simulink model "DSRCDOB"  (R2021a)
settings: Solver=VariableStepAuto  StartTime=0.0  StopTime=15.0  RelTol=1e-3
undefined symbols (not defined in the file): a, alpha, betac, delay, delay_a, gnet, omega
libraries: simulink x1
settings Model: Creator=shiva  LastModifiedBy=shiva

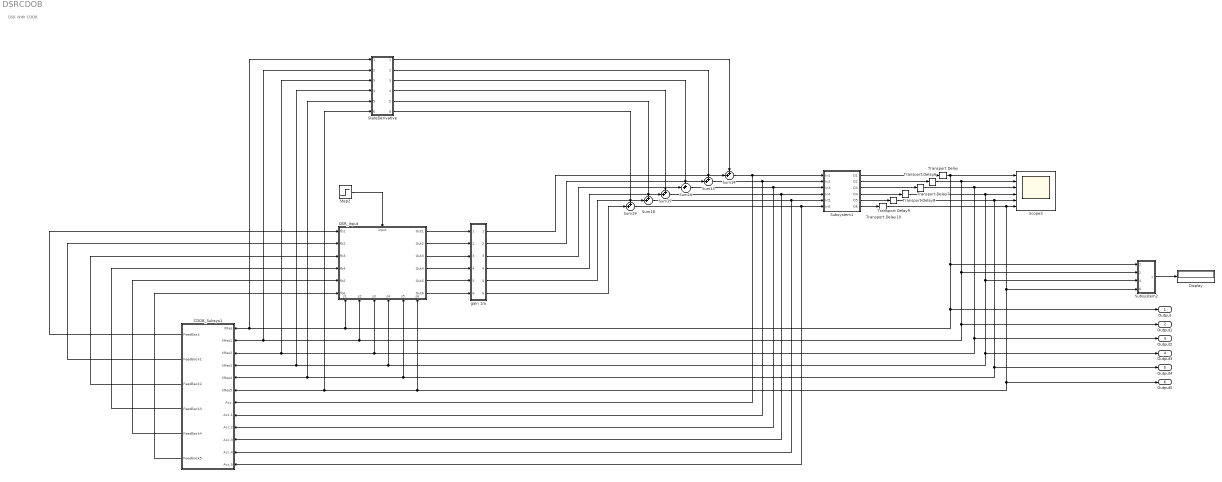
== system DSRCDOB ==
  note: DSR With CDOB
  CDOB_Subsys1 : Subsystem
  DSR_Input : Subsystem
      settings: PortSchema="{\"entries\":[{\"content\":{\"sides\":[{\"content\":{\"connectorIds\":[\"In1\",\"In2\",\"In3\",\"In4\",\"In5\",\"In6\"]},\"type\":\"ConnectorPlacement.EquallySpacedRectSide\",\"uuid\":\"7b8a38d4-2828-429e-a347-8750a0874c90\"},{\"content\":{\"connectorIds\":[\"Out1\",\"Out2\",\"Out3\",\"Out4\",\"Out5\",\"Out6\"],\"side\":\"RIGHT\"},\"type\":\"ConnectorPlacement.EquallySpacedRectSide\",\"uuid\":\"f1dcdaa7-0a93-43e2-be3b-ce942cee3b23\"},{\"content\":{\"connectorIds\":[\"In7\"],\"side\":\"TOP\"},\"type\":\"ConnectorPlacement.EquallySpacedRectSide\",\"uuid\":\"691a82b2-07cc-468b-b9a0-c0927a09fa47\"},{\"content\":{\"connectorIds\":[\"In8\",\"In9\",\"In10\",\"In11\",\"In12\",\"In13\"],\"side\":\"BOTTOM\"},\"type\":\"ConnectorPlacement.EquallySpacedRectSide\",\"uuid\":\"87ba8582-7e13-41cf-953e-972bab5f6463\"}]},\"type\":\"ConnectorPlacement.EquallySpacedConnector\",\"uuid\":\"6089c568-97aa-4e95-8448-5d1116d5973e\"}],\"packageUris\":[\"http://schema.mathworks.com/mf0/Connector/R2020b\"],\"version\":\"1.0\"}"
  Display : Display
  Scope3 : Scope  NumInputPorts=6
  StateDerivative : Subsystem
  Step2 : Step  Time=0  SampleTime=0
  Subsystem1 : Subsystem
  Subsystem2 : Subsystem
  Sum{14..19} (6 alike) : Sum  Inputs=++|
  Transport Delay{,6..10} (6 alike) : TransportDelay  DelayTime=delay_a
  gain 1/a : Subsystem
  Output : Outport
  Output1 : Outport  Port=2
  Output2 : Outport  Port=3
  Output3 : Outport  Port=4
  Output4 : Outport  Port=5
  Output5 : Outport  Port=6
  wires:
  Sum17/1 -> CDOB_Subsys1/10(Acc.3), Subsystem1/4(In4)
  Subsystem1/3(O3) -> Transport Delay7/1
  Step2/1 -> DSR_Input/7(input)
  Subsystem1/2(O2) -> Transport Delay6/1
  StateDerivative/5(Out5) -> Sum18/1
  StateDerivative/6(Out6) -> Sum19/1
  StateDerivative/1(Out1) -> Sum14/1
  StateDerivative/3(Out3) -> Sum16/1
  gain 1/a/1(Out1) -> Sum14/2
  Transport Delay6/1 -> Subsystem2/2(Input1), Output1/1, DSR_Input/9(s2), StateDerivative/2(Input1), CDOB_Subsys1/2(XRes1), Scope3/2
  DSR_Input/3(Out3) -> gain 1/a/3(In3)
  Transport Delay7/1 -> Output2/1, DSR_Input/10(s3), StateDerivative/3(Input2), CDOB_Subsys1/3(XRes2), Scope3/3
  CDOB_Subsys1/1(FeedBack) -> DSR_Input/1(fb1)
  Subsystem1/1(O1) -> Transport Delay/1
  Sum18/1 -> CDOB_Subsys1/11(Acc.4), Subsystem1/5(In5)
  DSR_Input/5(Out5) -> gain 1/a/5(In5)
  gain 1/a/4(Out4) -> Sum17/2
  CDOB_Subsys1/4(FeedBack3) -> DSR_Input/4(fb4)
  Transport Delay9/1 -> Output4/1, DSR_Input/12(s5), StateDerivative/5(Input4), CDOB_Subsys1/5(XRes4), Scope3/5
  Subsystem1/6(O6) -> Transport Delay10/1
  CDOB_Subsys1/2(FeedBack1) -> DSR_Input/2(fb2)
  DSR_Input/2(Out2) -> gain 1/a/2(In2)
  gain 1/a/2(Out2) -> Sum15/2
  CDOB_Subsys1/5(FeedBack4) -> DSR_Input/5(fb5)
  CDOB_Subsys1/3(FeedBack2) -> DSR_Input/3(fb3)
  Transport Delay10/1 -> Subsystem2/4(6), Output5/1, DSR_Input/13(s6), StateDerivative/6(Input5), CDOB_Subsys1/6(XRes5), Scope3/6
  StateDerivative/2(Out2) -> Sum15/1
  DSR_Input/4(Out4) -> gain 1/a/4(In4)
  DSR_Input/1(Out1) -> gain 1/a/1(In1)
  gain 1/a/3(Out3) -> Sum16/2
  Sum15/1 -> CDOB_Subsys1/8(Acc.1), Subsystem1/2(In2)
  DSR_Input/6(Out6) -> gain 1/a/6(In6)
  Subsystem1/5(O5) -> Transport Delay9/1
  gain 1/a/5(Out5) -> Sum18/2
  gain 1/a/6(Out6) -> Sum19/2
  StateDerivative/4(Out4) -> Sum17/1
  Transport Delay8/1 -> Subsystem2/3(4), Output3/1, DSR_Input/11(s4), StateDerivative/4(Input3), CDOB_Subsys1/4(XRes3), Scope3/4
  Subsystem1/4(O4) -> Transport Delay8/1
  Sum19/1 -> CDOB_Subsys1/12(Acc.5), Subsystem1/6(In6)
  Sum16/1 -> CDOB_Subsys1/9(Acc.2), Subsystem1/3(In3)
  Subsystem2/1(y) -> Display/1
  Sum14/1 -> CDOB_Subsys1/7(Acc.), Subsystem1/1(In1)
  CDOB_Subsys1/6(FeedBack5) -> DSR_Input/6(fb6)
  Transport Delay/1 -> Scope3/1, Subsystem2/1(Input), Output/1, DSR_Input/8(s1), StateDerivative/1(Input), CDOB_Subsys1/1(XRes)

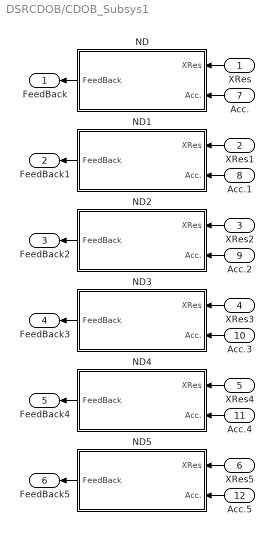
== system DSRCDOB/CDOB_Subsys1 ==
  XRes : Inport
  XRes1 : Inport  Port=2
  XRes2 : Inport  Port=3
  XRes3 : Inport  Port=4
  XRes4 : Inport  Port=5
  XRes5 : Inport  Port=6
  Acc. : Inport  Port=7
  Acc.1 : Inport  Port=8
  Acc.2 : Inport  Port=9
  Acc.3 : Inport  Port=10
  Acc.4 : Inport  Port=11
  Acc.5 : Inport  Port=12
  ND : Subsystem
  ND1 : Subsystem
  ND2 : Subsystem
  ND3 : Subsystem
  ND4 : Subsystem
  ND5 : Subsystem
  FeedBack : Outport
  FeedBack1 : Outport  Port=2
  FeedBack2 : Outport  Port=3
  FeedBack3 : Outport  Port=4
  FeedBack4 : Outport  Port=5
  FeedBack5 : Outport  Port=6
  wires:
  Acc./1 -> ND/2(Acc.)
  XRes/1 -> ND/1(XRes)
  Acc.4/1 -> ND4/2(Acc.)
  Acc.3/1 -> ND3/2(Acc.)
  XRes1/1 -> ND1/1(XRes)
  XRes2/1 -> ND2/1(XRes)
  XRes4/1 -> ND4/1(XRes)
  XRes5/1 -> ND5/1(XRes)
  Acc.2/1 -> ND2/2(Acc.)
  ND5/1(FeedBack) -> FeedBack5/1
  ND1/1(FeedBack) -> FeedBack1/1
  ND2/1(FeedBack) -> FeedBack2/1
  Acc.5/1 -> ND5/2(Acc.)
  ND4/1(FeedBack) -> FeedBack4/1
  ND/1(FeedBack) -> FeedBack/1
  ND3/1(FeedBack) -> FeedBack3/1
  XRes3/1 -> ND3/1(XRes)
  Acc.1/1 -> ND1/2(Acc.)

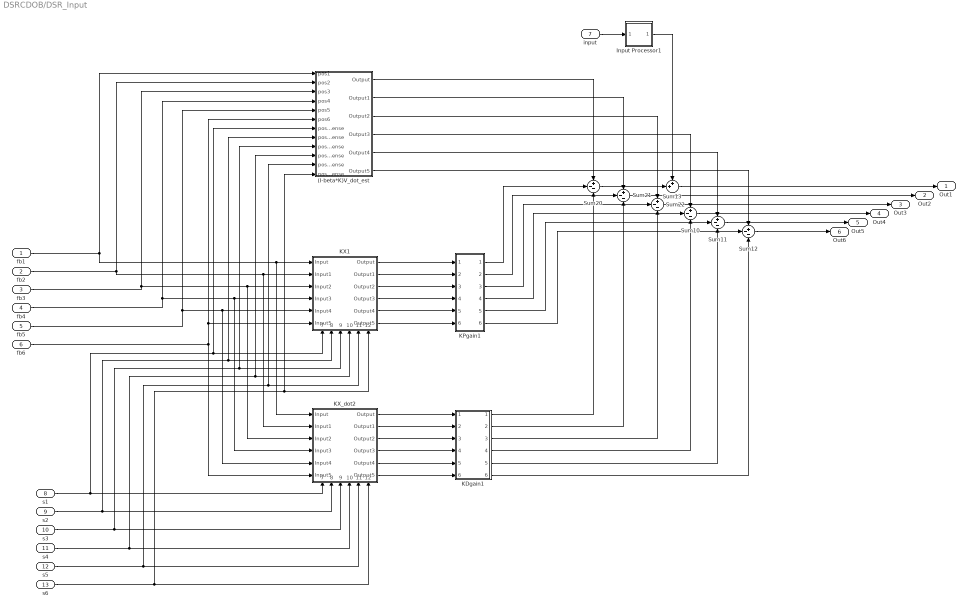
== system DSRCDOB/DSR_Input ==
  fb1 : Inport
  fb2 : Inport  Port=2
  fb3 : Inport  Port=3
  fb4 : Inport  Port=4
  fb5 : Inport  Port=5
  fb6 : Inport  Port=6
  input : Inport  Port=7
  s1 : Inport  Port=8
  s2 : Inport  Port=9
  s3 : Inport  Port=10
  s4 : Inport  Port=11
  s5 : Inport  Port=12
  s6 : Inport  Port=13
  (I-beta*K)V_dot_est : Subsystem
  Input Processor1 : Subsystem
  KDgain1 : Subsystem
  KPgain1 : Subsystem
  KX1 : Subsystem
      settings: PortSchema="{\"entries\":[{\"content\":{\"sides\":[{\"content\":{\"connectorIds\":[\"In1\",\"In2\",\"In3\",\"In4\",\"In5\",\"In6\"]},\"type\":\"ConnectorPlacement.EquallySpacedRectSide\",\"uuid\":\"24ff0189-2e26-4de2-9c90-2043606e3d63\"},{\"content\":{\"connectorIds\":[\"Out1\",\"Out2\",\"Out3\",\"Out4\",\"Out5\",\"Out6\"],\"side\":\"RIGHT\"},\"type\":\"ConnectorPlacement.EquallySpacedRectSide\",\"uuid\":\"7efe01dd-8101-429e-adc6-a10b45356e48\"},{\"content\":{\"connectorIds\":[],\"side\":\"TOP\"},\"type\":\"ConnectorPlacement.EquallySpacedRectSide\",\"uuid\":\"5c1fc1f4-b8b0-4afd-80fe-11f4d157d0fc\"},{\"content\":{\"connectorIds\":[\"In7\",\"In8\",\"In9\",\"In10\",\"In11\",\"In12\"],\"side\":\"BOTTOM\"},\"type\":\"ConnectorPlacement.EquallySpacedRectSide\",\"uuid\":\"e52c51d8-b236-4cc8-9958-a8d91e3741c4\"}]},\"type\":\"ConnectorPlacement.EquallySpacedConnector\",\"uuid\":\"3e3502e3-b8a3-4e9d-9b78-ab08dd870d4b\"}],\"packageUris\":[\"http://schema.mathworks.com/mf0/Connector/R2020b\"],\"version\":\"1.0\"}"
  KX_dot2 : Subsystem
      settings: PortSchema="{\"entries\":[{\"content\":{\"sides\":[{\"content\":{\"connectorIds\":[\"In1\",\"In2\",\"In3\",\"In4\",\"In5\",\"In6\"]},\"type\":\"ConnectorPlacement.EquallySpacedRectSide\",\"uuid\":\"24ff0189-2e26-4de2-9c90-2043606e3d63\"},{\"content\":{\"connectorIds\":[\"Out1\",\"Out2\",\"Out3\",\"Out4\",\"Out5\",\"Out6\"],\"side\":\"RIGHT\"},\"type\":\"ConnectorPlacement.EquallySpacedRectSide\",\"uuid\":\"7efe01dd-8101-429e-adc6-a10b45356e48\"},{\"content\":{\"connectorIds\":[],\"side\":\"TOP\"},\"type\":\"ConnectorPlacement.EquallySpacedRectSide\",\"uuid\":\"5c1fc1f4-b8b0-4afd-80fe-11f4d157d0fc\"},{\"content\":{\"connectorIds\":[\"In7\",\"In8\",\"In9\",\"In10\",\"In11\",\"In12\"],\"side\":\"BOTTOM\"},\"type\":\"ConnectorPlacement.EquallySpacedRectSide\",\"uuid\":\"bae418dc-ca78-4370-85bb-31cb43009c14\"}]},\"type\":\"ConnectorPlacement.EquallySpacedConnector\",\"uuid\":\"3e3502e3-b8a3-4e9d-9b78-ab08dd870d4b\"}],\"packageUris\":[\"http://schema.mathworks.com/mf0/Connector/R2020b\"],\"version\":\"1.0\"}"
  Sum{10..12,20..22} (6 alike) : Sum  Inputs=+--
  Sum13 : Sum  Inputs=++|
  Out1 : Outport
  Out2 : Outport  Port=2
  Out3 : Outport  Port=3
  Out4 : Outport  Port=4
  Out5 : Outport  Port=5
  Out6 : Outport  Port=6
  wires:
  KX_dot2/5(Output4) -> KDgain1/5(Output4)
  fb4/1 -> KX1/4(Input3), KX_dot2/4(Input3), (I-beta*K)V_dot_est/4(pos4)
  fb2/1 -> KX1/2(Input1), KX_dot2/2(Input1), (I-beta*K)V_dot_est/2(pos2)
  KDgain1/6(Out6) -> Sum12/3
  fb3/1 -> KX1/3(Input2), KX_dot2/3(Input2), (I-beta*K)V_dot_est/3(pos3)
  KPgain1/4(Out4) -> Sum10/2
  Sum10/1 -> Out4/1
  KPgain1/2(Out2) -> Sum21/2
  KX1/6(Output5) -> KPgain1/6(Output5)
  KX1/2(Output1) -> KPgain1/2(Output1)
  KPgain1/6(Out6) -> Sum12/2
  KX1/4(Output3) -> KPgain1/4(Output3)
  KX1/3(Output2) -> KPgain1/3(Output2)
  s6/1 -> KX_dot2/12(sense6), (I-beta*K)V_dot_est/12(pos6sense), KX1/12(sense6)
  KDgain1/4(Out4) -> Sum10/3
  fb5/1 -> KX1/5(Input4), KX_dot2/5(Input4), (I-beta*K)V_dot_est/5(pos5)
  Sum22/1 -> Out3/1
  Sum12/1 -> Out6/1
  KPgain1/3(Out3) -> Sum22/2
  KDgain1/5(Out5) -> Sum11/3
  KDgain1/2(Out2) -> Sum21/3
  s3/1 -> KX_dot2/9(sense3), (I-beta*K)V_dot_est/9(pos3sense), KX1/9(sense3)
  Sum20/1 -> Sum13/2
  KDgain1/3(Out3) -> Sum22/3
  KX_dot2/4(Output3) -> KDgain1/4(Output3)
  fb1/1 -> KX1/1(Input), KX_dot2/1(Input), (I-beta*K)V_dot_est/1(pos1)
  (I-beta*K)V_dot_est/1(Output) -> Sum20/1
  KX_dot2/6(Output5) -> KDgain1/6(Output5)
  s1/1 -> KX_dot2/7(sense1), (I-beta*K)V_dot_est/7(pos1sense), KX1/7(sense1)
  s5/1 -> KX_dot2/11(sense5), (I-beta*K)V_dot_est/11(pos5sense), KX1/11(sense5)
  KX_dot2/2(Output1) -> KDgain1/2(Output1)
  Sum21/1 -> Out2/1
  KPgain1/5(Out5) -> Sum11/2
  fb6/1 -> KX1/6(Input5), (I-beta*K)V_dot_est/6(pos6), KX_dot2/6(Input5)
  (I-beta*K)V_dot_est/3(Output2) -> Sum22/1
  s4/1 -> KX_dot2/10(sense4), (I-beta*K)V_dot_est/10(pos4sense), KX1/10(sense4)
  KX1/5(Output4) -> KPgain1/5(Output4)
  KDgain1/1(Out1) -> Sum20/3
  KX1/1(Output) -> KPgain1/1(Output)
  input/1 -> Input Processor1/1(Input)
  (I-beta*K)V_dot_est/2(Output1) -> Sum21/1
  KX_dot2/3(Output2) -> KDgain1/3(Output2)
  Sum11/1 -> Out5/1
  (I-beta*K)V_dot_est/4(Output3) -> Sum10/1
  KX_dot2/1(Output) -> KDgain1/1(Output)
  (I-beta*K)V_dot_est/5(Output4) -> Sum11/1
  (I-beta*K)V_dot_est/6(Output5) -> Sum12/1
  KPgain1/1(Out1) -> Sum20/2
  s2/1 -> KX_dot2/8(sense2), (I-beta*K)V_dot_est/8(pos2sense), KX1/8(sense2)
  Sum13/1 -> Out1/1
  Input Processor1/1(Out1) -> Sum13/1

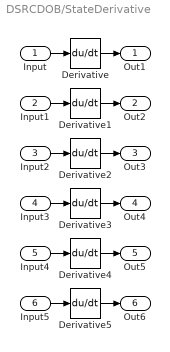
== system DSRCDOB/StateDerivative ==
  Input : Inport
  Input1 : Inport  Port=2
  Input2 : Inport  Port=3
  Input3 : Inport  Port=4
  Input4 : Inport  Port=5
  Input5 : Inport  Port=6
  Derivative{,1..5} (6 alike) : Derivative
  Out1 : Outport
  Out2 : Outport  Port=2
  Out3 : Outport  Port=3
  Out4 : Outport  Port=4
  Out5 : Outport  Port=5
  Out6 : Outport  Port=6
  wires:
  Input2/1 -> Derivative2/1
  Derivative1/1 -> Out2/1
  Derivative5/1 -> Out6/1
  Input/1 -> Derivative/1
  Input1/1 -> Derivative1/1
  Derivative4/1 -> Out5/1
  Input4/1 -> Derivative4/1
  Input3/1 -> Derivative3/1
  Derivative/1 -> Out1/1
  Input5/1 -> Derivative5/1
  Derivative2/1 -> Out3/1
  Derivative3/1 -> Out4/1

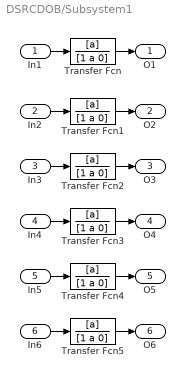
== system DSRCDOB/Subsystem1 ==
  In1 : Inport
  In2 : Inport  Port=2
  In3 : Inport  Port=3
  In4 : Inport  Port=4
  In5 : Inport  Port=5
  In6 : Inport  Port=6
  Transfer Fcn{,1..5} (6 alike) : TransferFcn  Numerator=[a]  Denominator=[1 a 0]
  O1 : Outport
  O2 : Outport  Port=2
  O3 : Outport  Port=3
  O4 : Outport  Port=4
  O5 : Outport  Port=5
  O6 : Outport  Port=6
  wires:
  Transfer Fcn1/1 -> O2/1
  In1/1 -> Transfer Fcn/1
  Transfer Fcn/1 -> O1/1
  In4/1 -> Transfer Fcn3/1
  Transfer Fcn3/1 -> O4/1
  In3/1 -> Transfer Fcn2/1
  In2/1 -> Transfer Fcn1/1
  Transfer Fcn2/1 -> O3/1
  Transfer Fcn5/1 -> O6/1
  In6/1 -> Transfer Fcn5/1
  In5/1 -> Transfer Fcn4/1
  Transfer Fcn4/1 -> O5/1

== system DSRCDOB/Subsystem2 ==
  Input : Inport
  Input1 : Inport  Port=2
  4 : Inport  Port=3
  6 : Inport  Port=4
  Abs : Abs
  Min : MinMax  Function=max  Inputs=3
  MinMax Running Resettable : simulink/Math Operations/MinMax Running Resettable  Function=max  vinit=0.0
  Sum7 : Sum  Inputs=|+-
  Sum8 : Sum  Inputs=|+-
  Sum9 : Sum  Inputs=|+-
  Zero : Constant  Value=0  OutDataTypeStr=Inherit: Inherit via back propagation
  y : Outport
  wires:
  Min/1 -> Abs/1
  6/1 -> Sum9/2
  Input/1 -> Sum7/1
  4/1 -> Sum8/2, Sum9/1
  Input1/1 -> Sum8/1, Sum7/2
  Sum8/1 -> Min/2
  Zero/1 -> MinMax Running Resettable/2
  Sum7/1 -> Min/1
  Abs/1 -> MinMax Running Resettable/1
  Sum9/1 -> Min/3
  MinMax Running Resettable/1 -> y/1

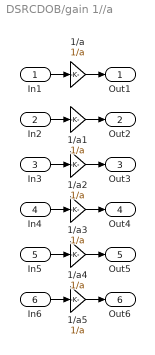
== system DSRCDOB/gain 1//a ==
  In1 : Inport
  In2 : Inport  Port=2
  In3 : Inport  Port=3
  In4 : Inport  Port=4
  In5 : Inport  Port=5
  In6 : Inport  Port=6
  1/a{,1..5} (6 alike) : Gain  Gain=1/a
  Out1 : Outport
  Out2 : Outport  Port=2
  Out3 : Outport  Port=3
  Out4 : Outport  Port=4
  Out5 : Outport  Port=5
  Out6 : Outport  Port=6
  wires:
  1/a2/1 -> Out3/1
  In1/1 -> 1/a/1
  In4/1 -> 1/a3/1
  1/a5/1 -> Out6/1
  In2/1 -> 1/a1/1
  1/a4/1 -> Out5/1
  1/a/1 -> Out1/1
  In6/1 -> 1/a5/1
  1/a3/1 -> Out4/1
  In5/1 -> 1/a4/1
  In3/1 -> 1/a2/1
  1/a1/1 -> Out2/1

== system DSRCDOB/CDOB_Subsys1/ND ==
  XRes : Inport
  Acc. : Inport  Port=2
  CDOB1 : Subsystem
  TimeDelayComp : Subsystem
  FeedBack : Outport
  wires:
  CDOB1/1(Dobsv) -> TimeDelayComp/2(Dobsv)
  Acc./1 -> CDOB1/2(Acc.)
  TimeDelayComp/1(FeedBack) -> FeedBack/1
  XRes/1 -> TimeDelayComp/1(SysOut), CDOB1/1(XRes)

== system DSRCDOB/CDOB_Subsys1/ND1 ==
  XRes : Inport
  Acc. : Inport  Port=2
  CDOB1 : Subsystem
  TimeDelayComp : Subsystem
  FeedBack : Outport
  wires:
  CDOB1/1(Dobsv) -> TimeDelayComp/2(Dobsv)
  Acc./1 -> CDOB1/2(Acc.)
  TimeDelayComp/1(FeedBack) -> FeedBack/1
  XRes/1 -> TimeDelayComp/1(SysOut), CDOB1/1(XRes)

== system DSRCDOB/CDOB_Subsys1/ND2 ==
  XRes : Inport
  Acc. : Inport  Port=2
  CDOB1 : Subsystem
  TimeDelayComp : Subsystem
  FeedBack : Outport
  wires:
  CDOB1/1(Dobsv) -> TimeDelayComp/2(Dobsv)
  Acc./1 -> CDOB1/2(Acc.)
  TimeDelayComp/1(FeedBack) -> FeedBack/1
  XRes/1 -> TimeDelayComp/1(SysOut), CDOB1/1(XRes)

== system DSRCDOB/CDOB_Subsys1/ND3 ==
  XRes : Inport
  Acc. : Inport  Port=2
  CDOB1 : Subsystem
  TimeDelayComp : Subsystem
  FeedBack : Outport
  wires:
  CDOB1/1(Dobsv) -> TimeDelayComp/2(Dobsv)
  Acc./1 -> CDOB1/2(Acc.)
  TimeDelayComp/1(FeedBack) -> FeedBack/1
  XRes/1 -> TimeDelayComp/1(SysOut), CDOB1/1(XRes)

== system DSRCDOB/CDOB_Subsys1/ND4 ==
  XRes : Inport
  Acc. : Inport  Port=2
  CDOB1 : Subsystem
  TimeDelayComp : Subsystem
  FeedBack : Outport
  wires:
  CDOB1/1(Dobsv) -> TimeDelayComp/2(Dobsv)
  Acc./1 -> CDOB1/2(Acc.)
  TimeDelayComp/1(FeedBack) -> FeedBack/1
  XRes/1 -> TimeDelayComp/1(SysOut), CDOB1/1(XRes)

== system DSRCDOB/CDOB_Subsys1/ND5 ==
  XRes : Inport
  Acc. : Inport  Port=2
  CDOB1 : Subsystem
  TimeDelayComp : Subsystem
  FeedBack : Outport
  wires:
  CDOB1/1(Dobsv) -> TimeDelayComp/2(Dobsv)
  Acc./1 -> CDOB1/2(Acc.)
  TimeDelayComp/1(FeedBack) -> FeedBack/1
  XRes/1 -> TimeDelayComp/1(SysOut), CDOB1/1(XRes)

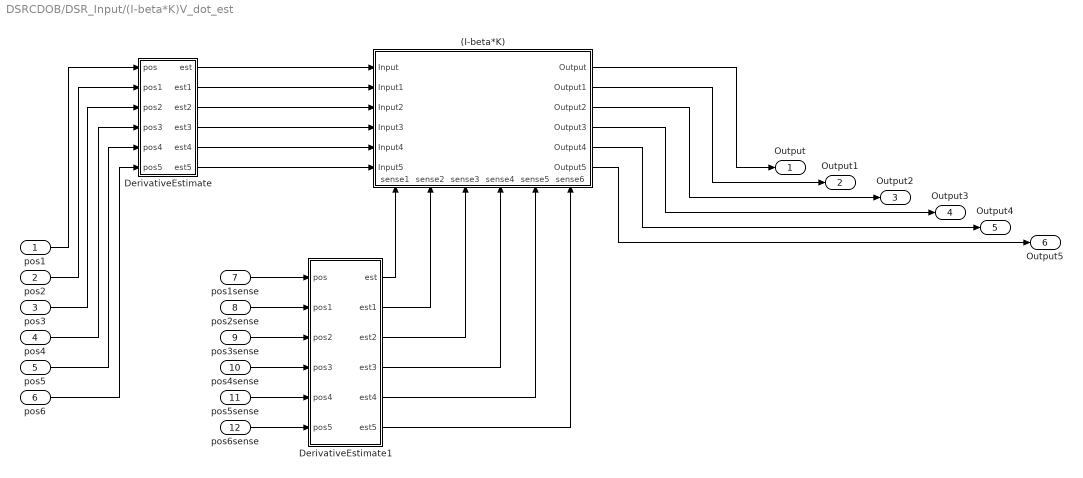
== system DSRCDOB/DSR_Input/(I-beta*K)V_dot_est ==
  pos1 : Inport
  pos2 : Inport  Port=2
  pos3 : Inport  Port=3
  pos4 : Inport  Port=4
  pos5 : Inport  Port=5
  pos6 : Inport  Port=6
  pos1sense : Inport  Port=7
  pos2sense : Inport  Port=8
  pos3sense : Inport  Port=9
  pos4sense : Inport  Port=10
  pos5sense : Inport  Port=11
  pos6sense : Inport  Port=12
  (I-beta*K) : Subsystem
      settings: PortSchema="{\"entries\":[{\"content\":{\"sides\":[{\"content\":{\"connectorIds\":[\"In1\",\"In2\",\"In3\",\"In4\",\"In5\",\"In6\"]},\"type\":\"ConnectorPlacement.EquallySpacedRectSide\",\"uuid\":\"24ff0189-2e26-4de2-9c90-2043606e3d63\"},{\"content\":{\"connectorIds\":[\"Out1\",\"Out2\",\"Out3\",\"Out4\",\"Out5\",\"Out6\"],\"side\":\"RIGHT\"},\"type\":\"ConnectorPlacement.EquallySpacedRectSide\",\"uuid\":\"7efe01dd-8101-429e-adc6-a10b45356e48\"},{\"content\":{\"connectorIds\":[],\"side\":\"TOP\"},\"type\":\"ConnectorPlacement.EquallySpacedRectSide\",\"uuid\":\"5c1fc1f4-b8b0-4afd-80fe-11f4d157d0fc\"},{\"content\":{\"connectorIds\":[\"In7\",\"In8\",\"In9\",\"In10\",\"In11\",\"In12\"],\"side\":\"BOTTOM\"},\"type\":\"ConnectorPlacement.EquallySpacedRectSide\",\"uuid\":\"be77b686-a0b8-400e-8c92-c0517b137255\"}]},\"type\":\"ConnectorPlacement.EquallySpacedConnector\",\"uuid\":\"3e3502e3-b8a3-4e9d-9b78-ab08dd870d4b\"}],\"packageUris\":[\"http://schema.mathworks.com/mf0/Connector/R2020b\"],\"version\":\"1.0\"}"
  DerivativeEstimate : Subsystem
  DerivativeEstimate1 : Subsystem
  Output : Outport
  Output1 : Outport  Port=2
  Output2 : Outport  Port=3
  Output3 : Outport  Port=4
  Output4 : Outport  Port=5
  Output5 : Outport  Port=6
  wires:
  DerivativeEstimate/3(est2) -> (I-beta*K)/3(Input2)
  DerivativeEstimate/6(est5) -> (I-beta*K)/6(Input5)
  pos2/1 -> DerivativeEstimate/2(pos1)
  DerivativeEstimate/4(est3) -> (I-beta*K)/4(Input3)
  DerivativeEstimate/2(est1) -> (I-beta*K)/2(Input1)
  DerivativeEstimate/1(est) -> (I-beta*K)/1(Input)
  DerivativeEstimate/5(est4) -> (I-beta*K)/5(Input4)
  (I-beta*K)/6(Output5) -> Output5/1
  (I-beta*K)/3(Output2) -> Output2/1
  (I-beta*K)/4(Output3) -> Output3/1
  (I-beta*K)/5(Output4) -> Output4/1
  pos5/1 -> DerivativeEstimate/5(pos4)
  pos6/1 -> DerivativeEstimate/6(pos5)
  pos3/1 -> DerivativeEstimate/3(pos2)
  (I-beta*K)/2(Output1) -> Output1/1
  pos1/1 -> DerivativeEstimate/1(pos)
  pos4/1 -> DerivativeEstimate/4(pos3)
  (I-beta*K)/1(Output) -> Output/1
  pos1sense/1 -> DerivativeEstimate1/1(pos)
  pos2sense/1 -> DerivativeEstimate1/2(pos1)
  pos3sense/1 -> DerivativeEstimate1/3(pos2)
  pos4sense/1 -> DerivativeEstimate1/4(pos3)
  pos5sense/1 -> DerivativeEstimate1/5(pos4)
  pos6sense/1 -> DerivativeEstimate1/6(pos5)
  DerivativeEstimate1/1(est) -> (I-beta*K)/7(sense1)
  DerivativeEstimate1/2(est1) -> (I-beta*K)/8(sense2)
  DerivativeEstimate1/3(est2) -> (I-beta*K)/9(sense3)
  DerivativeEstimate1/4(est3) -> (I-beta*K)/10(sense4)
  DerivativeEstimate1/5(est4) -> (I-beta*K)/11(sense5)
  DerivativeEstimate1/6(est5) -> (I-beta*K)/12(sense6)

== system DSRCDOB/DSR_Input/Input Processor1 ==
  Input : Inport
  Derivative : Derivative
  Gain : Gain  Gain=alpha
  Gain1 : Gain  Gain=2
  Sum : Sum  Inputs=|++
  inputGain : Gain  Gain=alpha*betac
  Out1 : Outport
  wires:
  Gain1/1 -> Sum/2
  Derivative/1 -> Gain1/1
  Input/1 -> Gain/1, Derivative/1
  Sum/1 -> inputGain/1
  Gain/1 -> Sum/1
  inputGain/1 -> Out1/1

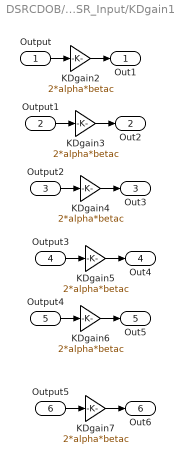
== system DSRCDOB/DSR_Input/KDgain1 ==
  Output : Inport
  Output1 : Inport  Port=2
  Output2 : Inport  Port=3
  Output3 : Inport  Port=4
  Output4 : Inport  Port=5
  Output5 : Inport  Port=6
  KDgain{2..7} (6 alike) : Gain  Gain=2*alpha*betac
  Out1 : Outport
  Out2 : Outport  Port=2
  Out3 : Outport  Port=3
  Out4 : Outport  Port=4
  Out5 : Outport  Port=5
  Out6 : Outport  Port=6
  wires:
  Output2/1 -> KDgain4/1
  KDgain4/1 -> Out3/1
  KDgain3/1 -> Out2/1
  KDgain6/1 -> Out5/1
  Output4/1 -> KDgain6/1
  Output/1 -> KDgain2/1
  KDgain2/1 -> Out1/1
  KDgain5/1 -> Out4/1
  Output3/1 -> KDgain5/1
  KDgain7/1 -> Out6/1
  Output5/1 -> KDgain7/1
  Output1/1 -> KDgain3/1

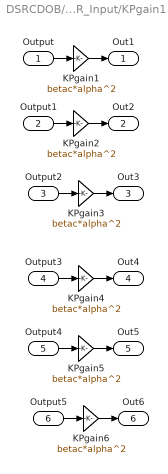
== system DSRCDOB/DSR_Input/KPgain1 ==
  Output : Inport
  Output1 : Inport  Port=2
  Output2 : Inport  Port=3
  Output3 : Inport  Port=4
  Output4 : Inport  Port=5
  Output5 : Inport  Port=6
  KPgain{1..6} (6 alike) : Gain  Gain=betac*alpha^2
  Out1 : Outport
  Out2 : Outport  Port=2
  Out3 : Outport  Port=3
  Out4 : Outport  Port=4
  Out5 : Outport  Port=5
  Out6 : Outport  Port=6
  wires:
  Output4/1 -> KPgain5/1
  KPgain1/1 -> Out1/1
  KPgain2/1 -> Out2/1
  KPgain5/1 -> Out5/1
  Output/1 -> KPgain1/1
  Output3/1 -> KPgain4/1
  Output5/1 -> KPgain6/1
  Output1/1 -> KPgain2/1
  KPgain3/1 -> Out3/1
  KPgain6/1 -> Out6/1
  Output2/1 -> KPgain3/1
  KPgain4/1 -> Out4/1

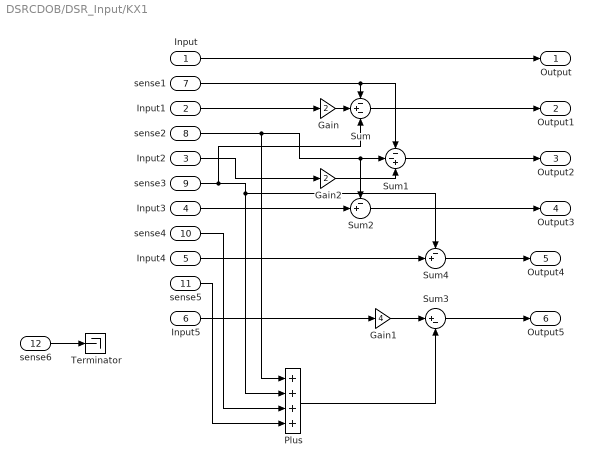
== system DSRCDOB/DSR_Input/KX1 ==
  Input : Inport
  Input1 : Inport  Port=2
  Input2 : Inport  Port=3
  Input3 : Inport  Port=4
  Input4 : Inport  Port=5
  Input5 : Inport  Port=6
  sense1 : Inport  Port=7
  sense2 : Inport  Port=8
  sense3 : Inport  Port=9
  sense4 : Inport  Port=10
  sense5 : Inport  Port=11
  sense6 : Inport  Port=12
  Gain : Gain  Gain=2
  Gain1 : Gain  Gain=4
  Gain2 : Gain  Gain=2
  Plus : Sum  Inputs=++++
  Sum : Sum  Inputs=-+-
  Sum1 : Sum  Inputs=--+
  Sum2 : Sum  Inputs=-+|
  Sum3 : Sum  Inputs=|+-
  Sum4 : Sum  Inputs=-+|
  Terminator : Terminator
  Output : Outport
  Output1 : Outport  Port=2
  Output2 : Outport  Port=3
  Output3 : Outport  Port=4
  Output4 : Outport  Port=5
  Output5 : Outport  Port=6
  wires:
  Input1/1 -> Gain/1
  Input/1 -> Output/1
  Input2/1 -> Gain2/1
  Sum1/1 -> Output2/1
  Input4/1 -> Sum4/2
  Gain/1 -> Sum/2
  Gain2/1 -> Sum1/3
  Sum/1 -> Output1/1
  Plus/1 -> Sum3/2
  Sum3/1 -> Output5/1
  Input5/1 -> Gain1/1
  Sum4/1 -> Output4/1
  Input3/1 -> Sum2/2
  Sum2/1 -> Output3/1
  Gain1/1 -> Sum3/1
  sense1/1 -> Sum1/1, Sum/1
  sense2/1 -> Sum2/1, Sum1/2, Plus/1
  sense3/1 -> Sum4/1, Plus/2, Sum/3
  sense4/1 -> Plus/3
  sense5/1 -> Plus/4
  sense6/1 -> Terminator/1

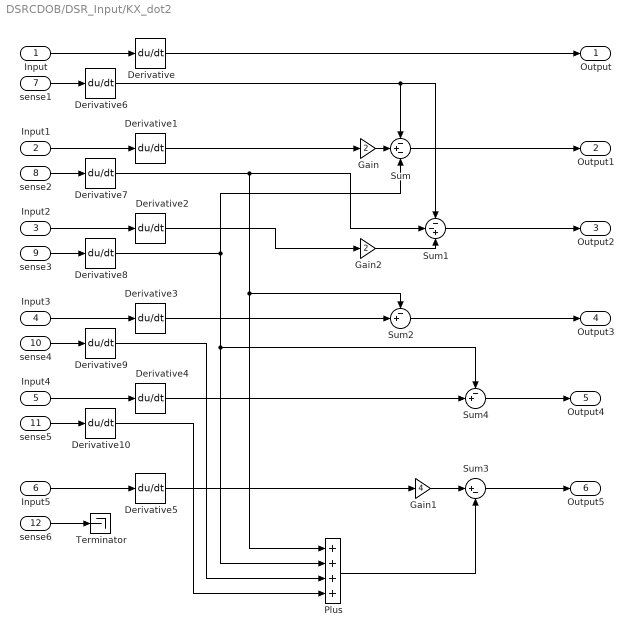
== system DSRCDOB/DSR_Input/KX_dot2 ==
  Input : Inport
  Input1 : Inport  Port=2
  Input2 : Inport  Port=3
  Input3 : Inport  Port=4
  Input4 : Inport  Port=5
  Input5 : Inport  Port=6
  sense1 : Inport  Port=7
  sense2 : Inport  Port=8
  sense3 : Inport  Port=9
  sense4 : Inport  Port=10
  sense5 : Inport  Port=11
  sense6 : Inport  Port=12
  Derivative{,1..10} (11 alike) : Derivative
  Gain : Gain  Gain=2
  Gain1 : Gain  Gain=4
  Gain2 : Gain  Gain=2
  Plus : Sum  Inputs=++++
  Sum : Sum  Inputs=-+-
  Sum1 : Sum  Inputs=--+
  Sum2 : Sum  Inputs=-+|
  Sum3 : Sum  Inputs=|+-
  Sum4 : Sum  Inputs=-+|
  Terminator : Terminator
  Output : Outport
  Output1 : Outport  Port=2
  Output2 : Outport  Port=3
  Output3 : Outport  Port=4
  Output4 : Outport  Port=5
  Output5 : Outport  Port=6
  wires:
  Input1/1 -> Derivative1/1
  Input/1 -> Derivative/1
  Input2/1 -> Derivative2/1
  Sum1/1 -> Output2/1
  Input4/1 -> Derivative4/1
  Gain/1 -> Sum/2
  Gain2/1 -> Sum1/3
  Sum/1 -> Output1/1
  Plus/1 -> Sum3/2
  Sum3/1 -> Output5/1
  Input5/1 -> Derivative5/1
  Sum4/1 -> Output4/1
  Input3/1 -> Derivative3/1
  Sum2/1 -> Output3/1
  Gain1/1 -> Sum3/1
  Derivative1/1 -> Gain/1
  Derivative2/1 -> Gain2/1
  Derivative3/1 -> Sum2/2
  Derivative4/1 -> Sum4/2
  Derivative5/1 -> Gain1/1
  sense1/1 -> Derivative6/1
  sense2/1 -> Derivative7/1
  sense3/1 -> Derivative8/1
  sense4/1 -> Derivative9/1
  sense5/1 -> Derivative10/1
  Derivative/1 -> Output/1
  Derivative6/1 -> Sum/1, Sum1/1
  Derivative7/1 -> Sum1/2, Sum2/1, Plus/1
  Derivative8/1 -> Sum4/1, Plus/2, Sum/3
  Derivative9/1 -> Plus/3
  Derivative10/1 -> Plus/4
  sense6/1 -> Terminator/1

== system DSRCDOB/CDOB_Subsys1/ND/CDOB1 ==
  XRes : Inport
  Acc. : Inport  Port=2
  Derivative : Derivative  CoefficientInTFapproximation=0
  Gain : Gain  Gain=gnet/a
  Sum : Sum  Inputs=-+|
  Sum8 : Sum  Inputs=+-+
  Transfer Fcn2 : TransferFcn  Numerator=[gnet]  Denominator=[1 gnet]
  Dobsv : Outport
  wires:
  Transfer Fcn2/1 -> Sum/2
  Sum8/1 -> Transfer Fcn2/1
  Derivative/1 -> Sum8/2, Gain/1
  Gain/1 -> Sum8/1, Sum/1
  Sum/1 -> Dobsv/1
  XRes/1 -> Derivative/1
  Acc./1 -> Sum8/3

== system DSRCDOB/CDOB_Subsys1/ND/TimeDelayComp ==
  SysOut : Inport
  Dobsv : Inport  Port=2
  DelayCom : TransferFcn  Numerator=[a]  Denominator=[1 a 0]
  Sum8 : Sum  Inputs=|++
  FeedBack : Outport
  wires:
  DelayCom/1 -> Sum8/2
  SysOut/1 -> Sum8/1
  Sum8/1 -> FeedBack/1
  Dobsv/1 -> DelayCom/1

== system DSRCDOB/CDOB_Subsys1/ND1/CDOB1 ==
  XRes : Inport
  Acc. : Inport  Port=2
  Derivative : Derivative  CoefficientInTFapproximation=0
  Gain : Gain  Gain=gnet/a
  Sum : Sum  Inputs=-+|
  Sum8 : Sum  Inputs=+-+
  Transfer Fcn2 : TransferFcn  Numerator=[gnet]  Denominator=[1 gnet]
  Dobsv : Outport
  wires:
  Transfer Fcn2/1 -> Sum/2
  Sum8/1 -> Transfer Fcn2/1
  Derivative/1 -> Sum8/2, Gain/1
  Gain/1 -> Sum8/1, Sum/1
  Sum/1 -> Dobsv/1
  XRes/1 -> Derivative/1
  Acc./1 -> Sum8/3

== system DSRCDOB/CDOB_Subsys1/ND1/TimeDelayComp ==
  SysOut : Inport
  Dobsv : Inport  Port=2
  DelayCom : TransferFcn  Numerator=[a]  Denominator=[1 a 0]
  Sum8 : Sum  Inputs=|++
  FeedBack : Outport
  wires:
  DelayCom/1 -> Sum8/2
  SysOut/1 -> Sum8/1
  Sum8/1 -> FeedBack/1
  Dobsv/1 -> DelayCom/1

== system DSRCDOB/CDOB_Subsys1/ND2/CDOB1 ==
  XRes : Inport
  Acc. : Inport  Port=2
  Derivative : Derivative  CoefficientInTFapproximation=0
  Gain : Gain  Gain=gnet/a
  Sum : Sum  Inputs=-+|
  Sum8 : Sum  Inputs=+-+
  Transfer Fcn2 : TransferFcn  Numerator=[gnet]  Denominator=[1 gnet]
  Dobsv : Outport
  wires:
  Transfer Fcn2/1 -> Sum/2
  Sum8/1 -> Transfer Fcn2/1
  Derivative/1 -> Sum8/2, Gain/1
  Gain/1 -> Sum8/1, Sum/1
  Sum/1 -> Dobsv/1
  XRes/1 -> Derivative/1
  Acc./1 -> Sum8/3

== system DSRCDOB/CDOB_Subsys1/ND2/TimeDelayComp ==
  SysOut : Inport
  Dobsv : Inport  Port=2
  DelayCom : TransferFcn  Numerator=[a]  Denominator=[1 a 0]
  Sum8 : Sum  Inputs=|++
  FeedBack : Outport
  wires:
  DelayCom/1 -> Sum8/2
  SysOut/1 -> Sum8/1
  Sum8/1 -> FeedBack/1
  Dobsv/1 -> DelayCom/1

== system DSRCDOB/CDOB_Subsys1/ND3/CDOB1 ==
  XRes : Inport
  Acc. : Inport  Port=2
  Derivative : Derivative  CoefficientInTFapproximation=0
  Gain : Gain  Gain=gnet/a
  Sum : Sum  Inputs=-+|
  Sum8 : Sum  Inputs=+-+
  Transfer Fcn2 : TransferFcn  Numerator=[gnet]  Denominator=[1 gnet]
  Dobsv : Outport
  wires:
  Transfer Fcn2/1 -> Sum/2
  Sum8/1 -> Transfer Fcn2/1
  Derivative/1 -> Sum8/2, Gain/1
  Gain/1 -> Sum8/1, Sum/1
  Sum/1 -> Dobsv/1
  XRes/1 -> Derivative/1
  Acc./1 -> Sum8/3

== system DSRCDOB/CDOB_Subsys1/ND3/TimeDelayComp ==
  SysOut : Inport
  Dobsv : Inport  Port=2
  DelayCom : TransferFcn  Numerator=[a]  Denominator=[1 a 0]
  Sum8 : Sum  Inputs=|++
  FeedBack : Outport
  wires:
  DelayCom/1 -> Sum8/2
  SysOut/1 -> Sum8/1
  Sum8/1 -> FeedBack/1
  Dobsv/1 -> DelayCom/1

== system DSRCDOB/CDOB_Subsys1/ND4/CDOB1 ==
  XRes : Inport
  Acc. : Inport  Port=2
  Derivative : Derivative  CoefficientInTFapproximation=0
  Gain : Gain  Gain=gnet/a
  Sum : Sum  Inputs=-+|
  Sum8 : Sum  Inputs=+-+
  Transfer Fcn2 : TransferFcn  Numerator=[gnet]  Denominator=[1 gnet]
  Dobsv : Outport
  wires:
  Transfer Fcn2/1 -> Sum/2
  Sum8/1 -> Transfer Fcn2/1
  Derivative/1 -> Sum8/2, Gain/1
  Gain/1 -> Sum8/1, Sum/1
  Sum/1 -> Dobsv/1
  XRes/1 -> Derivative/1
  Acc./1 -> Sum8/3

== system DSRCDOB/CDOB_Subsys1/ND4/TimeDelayComp ==
  SysOut : Inport
  Dobsv : Inport  Port=2
  DelayCom : TransferFcn  Numerator=[a]  Denominator=[1 a 0]
  Sum8 : Sum  Inputs=|++
  FeedBack : Outport
  wires:
  DelayCom/1 -> Sum8/2
  SysOut/1 -> Sum8/1
  Sum8/1 -> FeedBack/1
  Dobsv/1 -> DelayCom/1

== system DSRCDOB/CDOB_Subsys1/ND5/CDOB1 ==
  XRes : Inport
  Acc. : Inport  Port=2
  Derivative : Derivative  CoefficientInTFapproximation=0
  Gain : Gain  Gain=gnet/a
  Sum : Sum  Inputs=-+|
  Sum8 : Sum  Inputs=+-+
  Transfer Fcn2 : TransferFcn  Numerator=[gnet]  Denominator=[1 gnet]
  Dobsv : Outport
  wires:
  Transfer Fcn2/1 -> Sum/2
  Sum8/1 -> Transfer Fcn2/1
  Derivative/1 -> Sum8/2, Gain/1
  Gain/1 -> Sum8/1, Sum/1
  Sum/1 -> Dobsv/1
  XRes/1 -> Derivative/1
  Acc./1 -> Sum8/3

== system DSRCDOB/CDOB_Subsys1/ND5/TimeDelayComp ==
  SysOut : Inport
  Dobsv : Inport  Port=2
  DelayCom : TransferFcn  Numerator=[a]  Denominator=[1 a 0]
  Sum8 : Sum  Inputs=|++
  FeedBack : Outport
  wires:
  DelayCom/1 -> Sum8/2
  SysOut/1 -> Sum8/1
  Sum8/1 -> FeedBack/1
  Dobsv/1 -> DelayCom/1

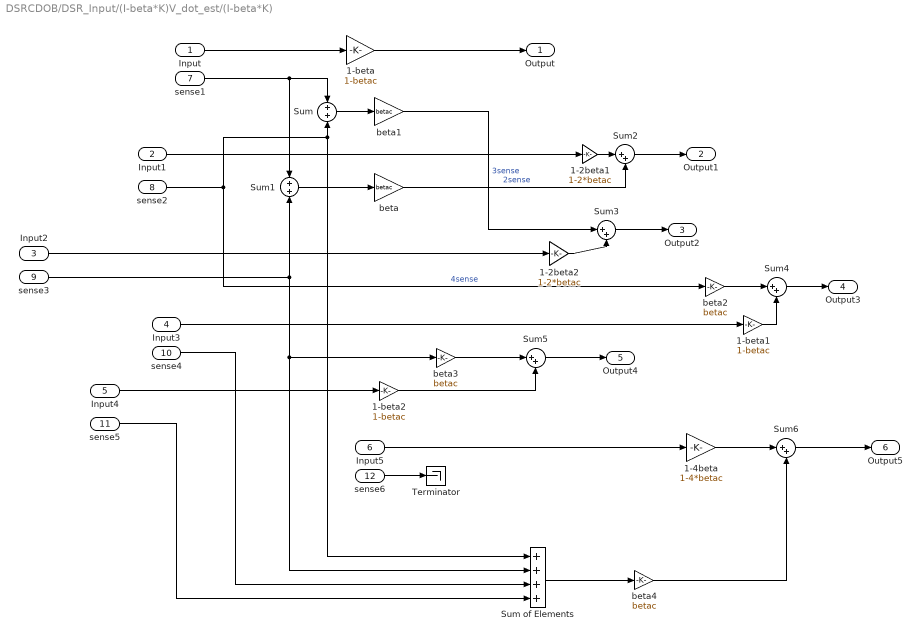
== system DSRCDOB/DSR_Input/(I-beta*K)V_dot_est/(I-beta*K) ==
  Input : Inport
  Input1 : Inport  Port=2
  Input2 : Inport  Port=3
  Input3 : Inport  Port=4
  Input4 : Inport  Port=5
  Input5 : Inport  Port=6
  sense1 : Inport  Port=7
  sense2 : Inport  Port=8
  sense3 : Inport  Port=9
  sense4 : Inport  Port=10
  sense5 : Inport  Port=11
  sense6 : Inport  Port=12
  1-2beta1 : Gain  Gain=1-2*betac
  1-2beta2 : Gain  Gain=1-2*betac
  1-4beta : Gain  Gain=1-4*betac
  1-beta : Gain  Gain=1-betac
  1-beta1 : Gain  Gain=1-betac
  1-beta2 : Gain  Gain=1-betac
  Sum : Sum  Inputs=+|+
  Sum of Elements : Sum  Inputs=++++
  Sum1 : Sum  Inputs=+|+
  Sum{2..6} (5 alike) : Sum  Inputs=|++
  Terminator : Terminator
  beta{,1..4} (5 alike) : Gain  Gain=betac
  Output : Outport
  Output1 : Outport  Port=2
  Output2 : Outport  Port=3
  Output3 : Outport  Port=4
  Output4 : Outport  Port=5
  Output5 : Outport  Port=6
  wires:
  Input/1 -> 1-beta/1
  1-2beta2/1 -> Sum3/2
  1-beta2/1 -> Sum5/2
  Sum4/1 -> Output3/1
  1-beta/1 -> Output/1
  beta/1 -> Sum2/2  "2sense"
  Sum6/1 -> Output5/1
  1-beta1/1 -> Sum4/2
  Input2/1 -> 1-2beta2/1
  1-2beta1/1 -> Sum2/1
  Input1/1 -> 1-2beta1/1
  beta4/1 -> Sum6/2
  Sum/1 -> beta1/1
  Input3/1 -> 1-beta1/1
  beta3/1 -> Sum5/1
  beta1/1 -> Sum3/1  "3sense"
  beta2/1 -> Sum4/1
  Sum5/1 -> Output4/1
  Input4/1 -> 1-beta2/1
  Sum1/1 -> beta/1
  1-4beta/1 -> Sum6/1
  Sum2/1 -> Output1/1
  Sum3/1 -> Output2/1
  Input5/1 -> 1-4beta/1
  Sum of Elements/1 -> beta4/1
  sense1/1 -> Sum1/1, Sum/1
  sense2/1 -> beta2/1, Sum of Elements/1, Sum/2  "4sense"
  sense3/1 -> beta3/1, Sum of Elements/2, Sum1/2
  sense5/1 -> Sum of Elements/4
  sense4/1 -> Sum of Elements/3
  sense6/1 -> Terminator/1

== system DSRCDOB/DSR_Input/(I-beta*K)V_dot_est/DerivativeEstimate ==
  pos : Inport
  pos1 : Inport  Port=2
  pos2 : Inport  Port=3
  pos3 : Inport  Port=4
  pos4 : Inport  Port=5
  pos5 : Inport  Port=6
  Derivative Estimator : Subsystem
  Derivative Estimator1 : Subsystem
  Derivative Estimator2 : Subsystem
  Derivative Estimator3 : Subsystem
  Derivative Estimator4 : Subsystem
  Derivative Estimator5 : Subsystem
  est : Outport
  est1 : Outport  Port=2
  est2 : Outport  Port=3
  est3 : Outport  Port=4
  est4 : Outport  Port=5
  est5 : Outport  Port=6
  wires:
  pos3/1 -> Derivative Estimator3/1(pos)
  Derivative Estimator4/1(est) -> est4/1
  Derivative Estimator2/1(est) -> est2/1
  Derivative Estimator3/1(est) -> est3/1
  Derivative Estimator1/1(est) -> est1/1
  pos1/1 -> Derivative Estimator1/1(pos)
  Derivative Estimator5/1(est) -> est5/1
  Derivative Estimator/1(est) -> est/1
  pos/1 -> Derivative Estimator/1(pos)
  pos2/1 -> Derivative Estimator2/1(pos)
  pos5/1 -> Derivative Estimator5/1(pos)
  pos4/1 -> Derivative Estimator4/1(pos)

== system DSRCDOB/DSR_Input/(I-beta*K)V_dot_est/DerivativeEstimate1 ==
  pos : Inport
  pos1 : Inport  Port=2
  pos2 : Inport  Port=3
  pos3 : Inport  Port=4
  pos4 : Inport  Port=5
  pos5 : Inport  Port=6
  Derivative Estimator : Subsystem
  Derivative Estimator1 : Subsystem
  Derivative Estimator2 : Subsystem
  Derivative Estimator3 : Subsystem
  Derivative Estimator4 : Subsystem
  Derivative Estimator5 : Subsystem
  est : Outport
  est1 : Outport  Port=2
  est2 : Outport  Port=3
  est3 : Outport  Port=4
  est4 : Outport  Port=5
  est5 : Outport  Port=6
  wires:
  pos3/1 -> Derivative Estimator3/1(pos)
  Derivative Estimator4/1(est) -> est4/1
  Derivative Estimator2/1(est) -> est2/1
  Derivative Estimator3/1(est) -> est3/1
  Derivative Estimator1/1(est) -> est1/1
  pos1/1 -> Derivative Estimator1/1(pos)
  Derivative Estimator5/1(est) -> est5/1
  Derivative Estimator/1(est) -> est/1
  pos/1 -> Derivative Estimator/1(pos)
  pos2/1 -> Derivative Estimator2/1(pos)
  pos5/1 -> Derivative Estimator5/1(pos)
  pos4/1 -> Derivative Estimator4/1(pos)

== system DSRCDOB/DSR_Input/(I-beta*K)V_dot_est/DerivativeEstimate/Derivative Estimator ==
  pos : Inport
  DSRdelay : Subsystem
  LPF : TransferFcn  Numerator=[omega^2]  Denominator=[delay^2 2*omega*delay^2 omega^2*delay^2]
  est : Outport
  wires:
  LPF/1 -> DSRdelay/1(Input)
  DSRdelay/1(Out1) -> est/1
  pos/1 -> LPF/1

== system DSRCDOB/DSR_Input/(I-beta*K)V_dot_est/DerivativeEstimate/Derivative Estimator1 ==
  pos : Inport
  DSRdelay : Subsystem
  LPF : TransferFcn  Numerator=[omega^2]  Denominator=[delay^2 2*omega*delay^2 omega^2*delay^2]
  est : Outport
  wires:
  LPF/1 -> DSRdelay/1(Input)
  DSRdelay/1(Out1) -> est/1
  pos/1 -> LPF/1

== system DSRCDOB/DSR_Input/(I-beta*K)V_dot_est/DerivativeEstimate/Derivative Estimator2 ==
  pos : Inport
  DSRdelay : Subsystem
  LPF : TransferFcn  Numerator=[omega^2]  Denominator=[delay^2 2*omega*delay^2 omega^2*delay^2]
  est : Outport
  wires:
  LPF/1 -> DSRdelay/1(Input)
  DSRdelay/1(Out1) -> est/1
  pos/1 -> LPF/1

== system DSRCDOB/DSR_Input/(I-beta*K)V_dot_est/DerivativeEstimate/Derivative Estimator3 ==
  pos : Inport
  DSRdelay : Subsystem
  LPF : TransferFcn  Numerator=[omega^2]  Denominator=[delay^2 2*omega*delay^2 omega^2*delay^2]
  est : Outport
  wires:
  LPF/1 -> DSRdelay/1(Input)
  DSRdelay/1(Out1) -> est/1
  pos/1 -> LPF/1

== system DSRCDOB/DSR_Input/(I-beta*K)V_dot_est/DerivativeEstimate/Derivative Estimator4 ==
  pos : Inport
  DSRdelay : Subsystem
  LPF : TransferFcn  Numerator=[omega^2]  Denominator=[delay^2 2*omega*delay^2 omega^2*delay^2]
  est : Outport
  wires:
  LPF/1 -> DSRdelay/1(Input)
  DSRdelay/1(Out1) -> est/1
  pos/1 -> LPF/1

== system DSRCDOB/DSR_Input/(I-beta*K)V_dot_est/DerivativeEstimate/Derivative Estimator5 ==
  pos : Inport
  DSRdelay : Subsystem
  LPF : TransferFcn  Numerator=[omega^2]  Denominator=[delay^2 2*omega*delay^2 omega^2*delay^2]
  est : Outport
  wires:
  LPF/1 -> DSRdelay/1(Input)
  DSRdelay/1(Out1) -> est/1
  pos/1 -> LPF/1

== system DSRCDOB/DSR_Input/(I-beta*K)V_dot_est/DerivativeEstimate1/Derivative Estimator ==
  pos : Inport
  DSRdelay : Subsystem
  LPF : TransferFcn  Numerator=[omega^2]  Denominator=[delay^2 2*omega*delay^2 omega^2*delay^2]
  est : Outport
  wires:
  LPF/1 -> DSRdelay/1(Input)
  DSRdelay/1(Out1) -> est/1
  pos/1 -> LPF/1

== system DSRCDOB/DSR_Input/(I-beta*K)V_dot_est/DerivativeEstimate1/Derivative Estimator1 ==
  pos : Inport
  DSRdelay : Subsystem
  LPF : TransferFcn  Numerator=[omega^2]  Denominator=[delay^2 2*omega*delay^2 omega^2*delay^2]
  est : Outport
  wires:
  LPF/1 -> DSRdelay/1(Input)
  DSRdelay/1(Out1) -> est/1
  pos/1 -> LPF/1

== system DSRCDOB/DSR_Input/(I-beta*K)V_dot_est/DerivativeEstimate1/Derivative Estimator2 ==
  pos : Inport
  DSRdelay : Subsystem
  LPF : TransferFcn  Numerator=[omega^2]  Denominator=[delay^2 2*omega*delay^2 omega^2*delay^2]
  est : Outport
  wires:
  LPF/1 -> DSRdelay/1(Input)
  DSRdelay/1(Out1) -> est/1
  pos/1 -> LPF/1

== system DSRCDOB/DSR_Input/(I-beta*K)V_dot_est/DerivativeEstimate1/Derivative Estimator3 ==
  pos : Inport
  DSRdelay : Subsystem
  LPF : TransferFcn  Numerator=[omega^2]  Denominator=[delay^2 2*omega*delay^2 omega^2*delay^2]
  est : Outport
  wires:
  LPF/1 -> DSRdelay/1(Input)
  DSRdelay/1(Out1) -> est/1
  pos/1 -> LPF/1

== system DSRCDOB/DSR_Input/(I-beta*K)V_dot_est/DerivativeEstimate1/Derivative Estimator4 ==
  pos : Inport
  DSRdelay : Subsystem
  LPF : TransferFcn  Numerator=[omega^2]  Denominator=[delay^2 2*omega*delay^2 omega^2*delay^2]
  est : Outport
  wires:
  LPF/1 -> DSRdelay/1(Input)
  DSRdelay/1(Out1) -> est/1
  pos/1 -> LPF/1

== system DSRCDOB/DSR_Input/(I-beta*K)V_dot_est/DerivativeEstimate1/Derivative Estimator5 ==
  pos : Inport
  DSRdelay : Subsystem
  LPF : TransferFcn  Numerator=[omega^2]  Denominator=[delay^2 2*omega*delay^2 omega^2*delay^2]
  est : Outport
  wires:
  LPF/1 -> DSRdelay/1(Input)
  DSRdelay/1(Out1) -> est/1
  pos/1 -> LPF/1

== system DSRCDOB/DSR_Input/(I-beta*K)V_dot_est/DerivativeEstimate/Derivative Estimator/DSRdelay ==
  Input : Inport
  Gain : Gain  Gain=2
  Sum : Sum  Inputs=-++
  Transport Delay1 : TransportDelay  DelayTime=2*delay
  Transport Delay2 : TransportDelay  DelayTime=delay
  Out1 : Outport
  wires:
  Input/1 -> Transport Delay2/1, Transport Delay1/1, Sum/2
  Transport Delay2/1 -> Gain/1
  Transport Delay1/1 -> Sum/3
  Gain/1 -> Sum/1
  Sum/1 -> Out1/1

== system DSRCDOB/DSR_Input/(I-beta*K)V_dot_est/DerivativeEstimate/Derivative Estimator1/DSRdelay ==
  Input : Inport
  Gain : Gain  Gain=2
  Sum : Sum  Inputs=-++
  Transport Delay1 : TransportDelay  DelayTime=2*delay
  Transport Delay2 : TransportDelay  DelayTime=delay
  Out1 : Outport
  wires:
  Input/1 -> Transport Delay2/1, Transport Delay1/1, Sum/2
  Transport Delay2/1 -> Gain/1
  Transport Delay1/1 -> Sum/3
  Gain/1 -> Sum/1
  Sum/1 -> Out1/1

== system DSRCDOB/DSR_Input/(I-beta*K)V_dot_est/DerivativeEstimate/Derivative Estimator2/DSRdelay ==
  Input : Inport
  Gain : Gain  Gain=2
  Sum : Sum  Inputs=-++
  Transport Delay1 : TransportDelay  DelayTime=2*delay
  Transport Delay2 : TransportDelay  DelayTime=delay
  Out1 : Outport
  wires:
  Input/1 -> Transport Delay2/1, Transport Delay1/1, Sum/2
  Transport Delay2/1 -> Gain/1
  Transport Delay1/1 -> Sum/3
  Gain/1 -> Sum/1
  Sum/1 -> Out1/1

== system DSRCDOB/DSR_Input/(I-beta*K)V_dot_est/DerivativeEstimate/Derivative Estimator3/DSRdelay ==
  Input : Inport
  Gain : Gain  Gain=2
  Sum : Sum  Inputs=-++
  Transport Delay1 : TransportDelay  DelayTime=2*delay
  Transport Delay2 : TransportDelay  DelayTime=delay
  Out1 : Outport
  wires:
  Input/1 -> Transport Delay2/1, Transport Delay1/1, Sum/2
  Transport Delay2/1 -> Gain/1
  Transport Delay1/1 -> Sum/3
  Gain/1 -> Sum/1
  Sum/1 -> Out1/1

== system DSRCDOB/DSR_Input/(I-beta*K)V_dot_est/DerivativeEstimate/Derivative Estimator4/DSRdelay ==
  Input : Inport
  Gain : Gain  Gain=2
  Sum : Sum  Inputs=-++
  Transport Delay1 : TransportDelay  DelayTime=2*delay
  Transport Delay2 : TransportDelay  DelayTime=delay
  Out1 : Outport
  wires:
  Input/1 -> Transport Delay2/1, Transport Delay1/1, Sum/2
  Transport Delay2/1 -> Gain/1
  Transport Delay1/1 -> Sum/3
  Gain/1 -> Sum/1
  Sum/1 -> Out1/1

== system DSRCDOB/DSR_Input/(I-beta*K)V_dot_est/DerivativeEstimate/Derivative Estimator5/DSRdelay ==
  Input : Inport
  Gain : Gain  Gain=2
  Sum : Sum  Inputs=-++
  Transport Delay1 : TransportDelay  DelayTime=2*delay
  Transport Delay2 : TransportDelay  DelayTime=delay
  Out1 : Outport
  wires:
  Input/1 -> Transport Delay2/1, Transport Delay1/1, Sum/2
  Transport Delay2/1 -> Gain/1
  Transport Delay1/1 -> Sum/3
  Gain/1 -> Sum/1
  Sum/1 -> Out1/1

== system DSRCDOB/DSR_Input/(I-beta*K)V_dot_est/DerivativeEstimate1/Derivative Estimator/DSRdelay ==
  Input : Inport
  Gain : Gain  Gain=2
  Sum : Sum  Inputs=-++
  Transport Delay1 : TransportDelay  DelayTime=2*delay
  Transport Delay2 : TransportDelay  DelayTime=delay
  Out1 : Outport
  wires:
  Input/1 -> Transport Delay2/1, Transport Delay1/1, Sum/2
  Transport Delay2/1 -> Gain/1
  Transport Delay1/1 -> Sum/3
  Gain/1 -> Sum/1
  Sum/1 -> Out1/1

== system DSRCDOB/DSR_Input/(I-beta*K)V_dot_est/DerivativeEstimate1/Derivative Estimator1/DSRdelay ==
  Input : Inport
  Gain : Gain  Gain=2
  Sum : Sum  Inputs=-++
  Transport Delay1 : TransportDelay  DelayTime=2*delay
  Transport Delay2 : TransportDelay  DelayTime=delay
  Out1 : Outport
  wires:
  Input/1 -> Transport Delay2/1, Transport Delay1/1, Sum/2
  Transport Delay2/1 -> Gain/1
  Transport Delay1/1 -> Sum/3
  Gain/1 -> Sum/1
  Sum/1 -> Out1/1

== system DSRCDOB/DSR_Input/(I-beta*K)V_dot_est/DerivativeEstimate1/Derivative Estimator2/DSRdelay ==
  Input : Inport
  Gain : Gain  Gain=2
  Sum : Sum  Inputs=-++
  Transport Delay1 : TransportDelay  DelayTime=2*delay
  Transport Delay2 : TransportDelay  DelayTime=delay
  Out1 : Outport
  wires:
  Input/1 -> Transport Delay2/1, Transport Delay1/1, Sum/2
  Transport Delay2/1 -> Gain/1
  Transport Delay1/1 -> Sum/3
  Gain/1 -> Sum/1
  Sum/1 -> Out1/1

== system DSRCDOB/DSR_Input/(I-beta*K)V_dot_est/DerivativeEstimate1/Derivative Estimator3/DSRdelay ==
  Input : Inport
  Gain : Gain  Gain=2
  Sum : Sum  Inputs=-++
  Transport Delay1 : TransportDelay  DelayTime=2*delay
  Transport Delay2 : TransportDelay  DelayTime=delay
  Out1 : Outport
  wires:
  Input/1 -> Transport Delay2/1, Transport Delay1/1, Sum/2
  Transport Delay2/1 -> Gain/1
  Transport Delay1/1 -> Sum/3
  Gain/1 -> Sum/1
  Sum/1 -> Out1/1

== system DSRCDOB/DSR_Input/(I-beta*K)V_dot_est/DerivativeEstimate1/Derivative Estimator4/DSRdelay ==
  Input : Inport
  Gain : Gain  Gain=2
  Sum : Sum  Inputs=-++
  Transport Delay1 : TransportDelay  DelayTime=2*delay
  Transport Delay2 : TransportDelay  DelayTime=delay
  Out1 : Outport
  wires:
  Input/1 -> Transport Delay2/1, Transport Delay1/1, Sum/2
  Transport Delay2/1 -> Gain/1
  Transport Delay1/1 -> Sum/3
  Gain/1 -> Sum/1
  Sum/1 -> Out1/1

== system DSRCDOB/DSR_Input/(I-beta*K)V_dot_est/DerivativeEstimate1/Derivative Estimator5/DSRdelay ==
  Input : Inport
  Gain : Gain  Gain=2
  Sum : Sum  Inputs=-++
  Transport Delay1 : TransportDelay  DelayTime=2*delay
  Transport Delay2 : TransportDelay  DelayTime=delay
  Out1 : Outport
  wires:
  Input/1 -> Transport Delay2/1, Transport Delay1/1, Sum/2
  Transport Delay2/1 -> Gain/1
  Transport Delay1/1 -> Sum/3
  Gain/1 -> Sum/1
  Sum/1 -> Out1/1
